simulink model "Test_Cart_Path_Logic_Flow_2019"  (R2019a)
settings: Solver=VariableStepAuto  StartTime=0.0  StopTime=stopTime  RelTol=1e-3
PreLoadFcn:
  | initializeParameters
InitFcn:
  | initializeParameters
StartFcn:
  | initializeParameters
undefined symbols (not defined in the file): bale, baleParam, cart, cartParam, contactGripper, floorParam, manip, TsCtrl, X, Y, Z
libraries: sm_lib x216, nesl_utility x30, fl_lib x4, robotcorelib x2, robotmaniplib x2, simulink x2, Multibody_Multiphysics_Lib x2
(part 6 of 6)

== system Test_Cart_Path_Logic_Flow_2019/Subsystem/Position Actuated Robot Environment1/Mobile Robot/Right_Wheel/tire_full_4 ==
  Inertia : sm_lib/Body Elements/Inertia  InertiaType=Custom  Mass=17.8326781714329  MassUnits=kg  CenterOfMass=[0, 0, 0]  CenterOfMassUnits=m  MomentsOfInertia=[0.6913557394867444, 0.6913966993638616, 1.203079850798329]  MomentsOfInertiaUnits=kg*m^2  ProductsOfInertia=[4.794651980616825e-06, -1.915933556339341e-05, 1.097804687661671e-05]  ProductsOfInertiaUnits=kg*m^2  GraphicType=None  MarkerShape=Inertia  MarkerSize=20  GraphicVisPropType=SimpleVisualProperties  GraphicDiffuseColor=[0.5 0.5 0.5]  GraphicSpecularColor=[0.5 0.5 0.5 1.0]  GraphicAmbientColor=[0.15 0.15 0.15 1.0]  GraphicEmissiveColor=[0.0 0.0 0.0 1.0]  GraphicShininess=75  GraphicOpacity=1.0
  InertiaOriginTransform : sm_lib/Frames and Transforms/Rigid Transform  TranslationMethod=Cartesian  TranslationStandardOffset=0  TranslationStandardOffsetUnits=m  TranslationStandardAxis=+Z  TranslationCartesianOffset=[2.008717404642495e-05, -5.178921586005947e-06, -0.02748439675177222]  TranslationCartesianOffsetUnits=m  TranslationROffset=0  TranslationROffsetUnits=m  TranslationZOffset=0  TranslationZOffsetUnits=m  TranslationThetaOffset=0  TranslationThetaOffsetUnits=deg  RotationMethod=RotationSequence  RotationAngleUnits=deg  RotationStandardAxis=+Z  RotationAngle=0.0  RotationArbitraryAxis=[0 0 1]  FollAlignAxisA=+X  BaseAlignAxisA=+Y  FollAlignAxisB=+Y  BaseAlignAxisB=+Z  RotationSequenceAxes=BaseAxes  RotationSequence=XYZ  RotationSequenceAngles=[0, 0, 0]  RotationSequenceAnglesUnits=rad  RotationMatrix=[1 0 0; 0 1 0; 0 0 1]  Quaternion=[1 0 0 0]
  ReferenceFrame : sm_lib/Frames and Transforms/Reference Frame
  Visual : sm_lib/Body Elements/File Solid  ExtGeomFileName=/tire_coupling.stl  UnitType=Custom  ExtGeomFileUnits=m  StepReaderType=HEX  ExportConvexHullGeometry=off  InertiaType=Custom  Mass=0  MassUnits=kg  CenterOfMass=[0, 0, 0]  CenterOfMassUnits=m  MomentsOfInertia=[0, 0, 0]  MomentsOfInertiaUnits=kg*m^2  ProductsOfInertia=[0, 0, 0]  ProductsOfInertiaUnits=kg*m^2  BasedOnType=DensityFromFile  Density=1000  DensityUnits=kg/m^3  DoExposeReferenceFrame=on  SerializedFrames=<Frames/>  GraphicType=FromGeometry  MarkerShape=Sphere  MarkerSize=10  GraphicVisPropType=SimpleVisualProperties  GraphicDiffuseColor=[0.792156862745098, 0.8196078431372549, 0.9333333333333333]  GraphicSpecularColor=[0.5 0.5 0.5 1.0]  GraphicAmbientColor=[0.15 0.15 0.15 1.0]  GraphicEmissiveColor=[0.0 0.0 0.0 1.0]  GraphicShininess=75  GraphicOpacity=1
  Visual1 : sm_lib/Body Elements/File Solid  ExtGeomFileName=/tire.stl  UnitType=Custom  ExtGeomFileUnits=m  StepReaderType=HEX  ExportConvexHullGeometry=off  InertiaType=Custom  Mass=0  MassUnits=kg  CenterOfMass=[0, 0, 0]  CenterOfMassUnits=m  MomentsOfInertia=[0, 0, 0]  MomentsOfInertiaUnits=kg*m^2  ProductsOfInertia=[0, 0, 0]  ProductsOfInertiaUnits=kg*m^2  BasedOnType=DensityFromFile  Density=1000  DensityUnits=kg/m^3  DoExposeReferenceFrame=on  SerializedFrames=<Frames/>  GraphicType=FromGeometry  MarkerShape=Sphere  MarkerSize=10  GraphicVisPropType=SimpleVisualProperties  GraphicDiffuseColor=[0.4117647058823529, 0.4117647058823529, 0.4156862745098039]  GraphicSpecularColor=[0.5 0.5 0.5 1.0]  GraphicAmbientColor=[0.15 0.15 0.15 1.0]  GraphicEmissiveColor=[0.0 0.0 0.0 1.0]  GraphicShininess=75  GraphicOpacity=1
  VisualOrigin1Transform : sm_lib/Frames and Transforms/Rigid Transform  TranslationMethod=Cartesian  TranslationStandardOffset=0  TranslationStandardOffsetUnits=m  TranslationStandardAxis=+Z  TranslationCartesianOffset=[-0.2286256789738323, -0.1469884823979781, 0.06636411353729821]  TranslationCartesianOffsetUnits=m  TranslationROffset=0  TranslationROffsetUnits=m  TranslationZOffset=0  TranslationZOffsetUnits=m  TranslationThetaOffset=0  TranslationThetaOffsetUnits=deg  RotationMethod=RotationSequence  RotationAngleUnits=deg  RotationStandardAxis=+Z  RotationAngle=0.0  RotationArbitraryAxis=[0 0 1]  FollAlignAxisA=+X  BaseAlignAxisA=+Y  FollAlignAxisB=+Y  BaseAlignAxisB=+Z  RotationSequenceAxes=BaseAxes  RotationSequence=XYZ  RotationSequenceAngles=[0.3764958615785354, -1.570796326794896, 0]  RotationSequenceAnglesUnits=rad  RotationMatrix=[1 0 0; 0 1 0; 0 0 1]  Quaternion=[1 0 0 0]
  VisualOriginTransform : sm_lib/Frames and Transforms/Rigid Transform  TranslationMethod=Cartesian  TranslationStandardOffset=0  TranslationStandardOffsetUnits=m  TranslationStandardAxis=+Z  TranslationCartesianOffset=[-1.89873840045938, -0.3026283430274336, -0.01269999999999993]  TranslationCartesianOffsetUnits=m  TranslationROffset=0  TranslationROffsetUnits=m  TranslationZOffset=0  TranslationZOffsetUnits=m  TranslationThetaOffset=0  TranslationThetaOffsetUnits=deg  RotationMethod=RotationSequence  RotationAngleUnits=deg  RotationStandardAxis=+Z  RotationAngle=0.0  RotationArbitraryAxis=[0 0 1]  FollAlignAxisA=+X  BaseAlignAxisA=+Y  FollAlignAxisB=+Y  BaseAlignAxisB=+Z  RotationSequenceAxes=BaseAxes  RotationSequence=XYZ  RotationSequenceAngles=[6.351795451943518e-33, -1.084878189679438e-32, -2.465190328815419e-32]  RotationSequenceAnglesUnits=rad  RotationMatrix=[1 0 0; 0 1 0; 0 0 1]  Quaternion=[1 0 0 0]
  x4_AxisInvTransform : sm_lib/Frames and Transforms/Rigid Transform  TranslationMethod=Cartesian  TranslationStandardOffset=0  TranslationStandardOffsetUnits=m  TranslationStandardAxis=+Z  TranslationCartesianOffset=[0, 0, 0]  TranslationCartesianOffsetUnits=m  TranslationROffset=0  TranslationROffsetUnits=m  TranslationZOffset=0  TranslationZOffsetUnits=m  TranslationThetaOffset=0  TranslationThetaOffsetUnits=deg  RotationMethod=ArbitraryAxis  RotationAngleUnits=rad  RotationStandardAxis=+Z  RotationAngle=0  RotationArbitraryAxis=[1, 0, 0]  FollAlignAxisA=+X  BaseAlignAxisA=+Y  FollAlignAxisB=+Y  BaseAlignAxisB=+Z  RotationSequenceAxes=FollowerAxes  RotationSequence=XYX  RotationSequenceAngles=[0 0 0]  RotationSequenceAnglesUnits=deg  RotationMatrix=[1 0 0; 0 1 0; 0 0 1]  Quaternion=[1 0 0 0]
  F : PMIOPort  Side=Left
  connections:
  Inertia/RConn1 -- InertiaOriginTransform/RConn1
  InertiaOriginTransform/LConn1 -- ReferenceFrame/RConn1 -- VisualOrigin1Transform/LConn1 -- VisualOriginTransform/LConn1 -- x4_AxisInvTransform/LConn1
  Visual/RConn1 -- VisualOriginTransform/RConn1
  Visual1/RConn1 -- VisualOrigin1Transform/RConn1
  x4_AxisInvTransform/RConn1 -- F/RConn1

== matlab function Test_Cart_Path_Logic_Flow_2019/Subsystem/Cart Inverse Kinematics1/cartTraj2Signal/cartTraj2Signal ==
  data: u input; w_r output; r input; b input; w_l output
function [w_r, w_l] = cartTraj2Signal(u,r,b)
w_r=((2*u(1)/r)+(u(2)*b/r))/2;
w_l=(2*u(1)/r)-w_r;
end

== matlab function Test_Cart_Path_Logic_Flow_2019/Subsystem/Position Actuated Robot Environment1/Mobile Robot/Cart Forward Kinematics/cartSignal2Traj/cartSignal2Traj ==
  data: u input; v output; r input; b input; w output
function [v,w] = cartSignal2Traj(u,r,b)
v=r*(u(1)+u(2))/2;
w=r*(u(1)-u(2))/b;
end

== stateflow chart Test_Cart_Path_Logic_Flow_2019/Supervisory Logic ==
  settings: updateMethod=DISCRETE  sampleTime=TsWaypoint
  state ManipulatorMotion [parallel]
    settings: executionOrder=2
    state StepOnManipTrajectory
      entry:
      currentManipState=currentManipState+1;
    state InTransition_M
    state SetManipConfiguration
      entry,during:
      targetManipPos=manipTrajectory(:,currentManipState);
      manipPosDiff=abs(manipCurrPose-manipTrajectory(:,currentManipState));
    state CheckForManipWaypoint
      entry:Gripper.SetGrip
      if currentManipTarget < size(manipWayPoints,2)
      currentManipTarget=currentManipTarget+1;
      end
    (default) -> InTransition_M : {currentManipState=1;
        | currentManipTarget=1;}
    SetManipConfiguration -> InTransition_M [order 1] : [currentManipTarget == size(manipWayPoints,2) || ~checkManip]
        | {MobileMotion.Moved;}
    InTransition_M -> SetManipConfiguration : Move
    StepOnManipTrajectory -> SetManipConfiguration
    SetManipConfiguration -> StepOnManipTrajectory [order 3] : [checkStateTolerance("Manip")]
    SetManipConfiguration -> CheckForManipWaypoint [order 2] : [checkWaypointTolerance("Manip")]
    CheckForManipWaypoint -> SetManipConfiguration : GripSet
  state Gripper [parallel]
    settings: executionOrder=3
    state InTransition_G
    state CloseGripper
      entry:
      gripCmd=1;
    state OpenGripper
      entry:
      gripCmd=-1;
    (default) -> InTransition_G
    (junction 86) -> InTransition_G
    (junction 78) -> InTransition_G
    CloseGripper -> (junction 86) : [after(0.5,sec)]
        | {ManipulatorMotion.GripSet;}
    OpenGripper -> (junction 78) : [after(0.5,sec)]
        | {ManipulatorMotion.GripSet;}
    InTransition_G -> (junction 75) : SetGrip
    (junction 75) -> OpenGripper [order 2]
    (junction 75) -> CloseGripper [order 1] : [checkGrip]
  state MobileMotion [parallel]
    settings: executionOrder=1
    state StepOnMobileTrajectory
      entry:
      currentMobileState=currentMobileState+1;
    state SetMobileConfiguration
      entry,during:
      targetMobilePos=mobileTrajectory(:,currentMobileState);
      mobilePosDiff=abs(mobileCurrPose-mobileTrajectory([1 2 4],currentMobileState));
    state CheckForMobileWaypoint
      entry:ManipulatorMotion.Move
      if currentMobileTarget < size(mobileWayPoints,2)
      currentMobileTarget=currentMobileTarget+1;
      end
    StepOnMobileTrajectory -> SetMobileConfiguration
    SetMobileConfiguration -> StepOnMobileTrajectory [order 2] : [checkStateTolerance("Mobile")]
    (default) -> SetMobileConfiguration : {currentMobileState=1;
        | currentMobileTarget=1;}
    SetMobileConfiguration -> CheckForMobileWaypoint [order 1] : [checkWaypointTolerance("Mobile")]
    CheckForMobileWaypoint -> SetMobileConfiguration : Moved
  data: atWaypoint function_output; select function_input; move function_output; grip function_output; atState function_output; select function_input; gripCmd output double size=1; gripForce input; manipTrajectory input; manipCurrPose input; mobileTrajectory input; mobileCurrPose input; mobileWayPoints input; manipWayPoints input; targetManipPos output; manipPosDiff output; mobilePosDiff output; currentManipState local; currentMobileState local; currentMobileTarget local; currentManipTarget local; targetMobilePos output; manipTolerance input; mobileTolerance input
  events: GripSet local FUNCTION_CALL_EVENT; Move local FUNCTION_CALL_EVENT; SetGrip local FUNCTION_CALL_EVENT; Moved local FUNCTION_CALL_EVENT
  function atWaypoint = checkWaypointTolerance(select):
    | function atWaypoint = checkWaypointTolerance(select)
    | % Checks if a waypoint has been reached within tolerance
    | 
    | if select=="Manip"
    |     reachedWaypoint = all(abs(manipCurrPose-manipWayPoints(1:6,currentManipTarget)) < manipTolerance);
    |     atWaypoint = reachedWaypoint && currentManipTarget <= size(manipWayPoints,2);
    | 
    | elseif select=="Mobile"
    |     reachedWaypoint = all(abs(mobileCurrPose(1:2)-mobileWayPoints(1:2,currentMobileTarget)) < mobileTolerance);
    |     atWaypoint = reachedWaypoint && currentMobileTarget <= size(mobileWayPoints,2);
    | end
    | 
    | end
  function move = checkManip:
    | function move = checkManip
    | % Checks the presence of a bale based on a minimum force threshold
    | 
    | move = mobileWayPoints(3, currentMobileTarget);
    | 
    | end
  function grip = checkGrip:
    | function grip = checkGrip
    | % Returns the grip status (0 or 1) at the current waypoint
    | 
    | grip = manipWayPoints(7,currentManipTarget);
    |  
    | end
  function atState = checkStateTolerance(select):
    | function atState = checkStateTolerance(select)
    | % Check if a robot state has been reached within tolerance
    | 
    | if select=="Manip"
    |     reachedPoint = all(abs(manipCurrPose-manipTrajectory(:,currentManipState)) < manipTolerance);
    |     atState = reachedPoint && currentManipState < size(manipTrajectory,2);
    | 
    | elseif select=="Mobile"
    |     reachedPoint = all(abs(mobileCurrPose-mobileTrajectory([1 2 4],currentMobileState)) < mobileTolerance);
    |     atState = reachedPoint && currentMobileState < size(mobileTrajectory,2);
    | end
    | 
    | end
